simulink model "cpu1"  (R2022b)
settings: Solver=FixedStepDiscrete  StartTime=0.0  StopTime=Inf  RelTol=1e-3  EnableMultiTasking=on
model workspace (MAT data in the model file):
  x = 1
undefined symbols (not defined in the file): C28x, CPU1, CPU2, EALLOW, EDIS
libraries: c2837xDlib x11, dspstat3 x5, c280xlib x4, slpidlib x2, c2802xlib x2, svdutilitieslib x1, dspswit3 x1, idelinklib_common x1
(part 2 of 2)

== matlab function cpu1/Subsystem1/MATLAB Function2 ==
  data: pot_value input; enc input; first_range output; center input; a input; offset input
function first_range = fcn(pot_value,enc,center,a,offset)

    x = center+offset;
    if pot_value < x-(2*a)
        %transition = [-2, -2];
        first_range = -2;
        return
    elseif pot_value < x-a
        transition = [-2, -1];
    elseif pot_value < x
        transition = [-1, 0];
    elseif pot_value < x+a
        transition = [0, 1];
    elseif pot_value < x+(2*a)
        transition = [1, 2];
    else
        %transition = [2, 2];
        first_range = 2;
        return
    end
    distances = abs((x+transition*a)-pot_value);
    if distances(1) <= distances(2)
        index = 1;
    else
        index = 2;
    end
    if distances(index) < 130
        first_range = transition(index);
        return
    end
    %if index == 1
    if enc > 0
        first_range = transition(1);
    else
        first_range = transition(2);
    end
%     else
%         if enc > 0
%             first_range = transition(1);
%         else
%             first_range = transition(2);
%         end

== stateflow chart cpu1/Subsystem/saturation tuned ==
  state state13
    sat = double(delta);
    kp= 0.35;
    if (abs(delta)<=0.5)
    ki=0.18;
    else
    ki=0.12;
    end
    reset = 1;
  state state12
    if delta > 0
    sat = 1;
    else
    sat = -1;
    end
    kp= 0.25;
    reset =0;
  state init
    f20 = 0;
    f15 = 0;
    f10 = 0;
    kp = 0;
    ki = 0;
    kd = 0;
    sat = 0;
  state else
    kp=0;
    sat=0;
    reset =1;
  state state10
    if delta > 0
    sat = 5;
    else
    sat = -5;
    end
    if f20 == 1 && f15==1 && f10==1
    kp = 0.07;
    elseif f20==0 && f15==1 && f10==1
    kp = 0.08;
    elseif f20==0 && f15==0 && f10==1
    kp = 0.08;
    else
    kp= 0.09;
    end
    reset =0;
  state state1
    if delta > 0
    sat = 20;
    else
    sat = -20;
    end
    kp = 0.025;
    f20 = 1;
    reset=0;
  state state9
    if delta > 0
    sat = 15;
    else
    sat = -15;
    end
    if f20 == 1
    kp = 0.03;
    else
    kp = 0.0334;
    end
    f15 = 1;
    reset=0;
  state state8
    if delta > 0
    sat = 10;
    else
    sat = -10;
    end
    if f20 == 1 && f15==1
    kp = 0.04;
    elseif f15==1 && f20==0
    kp = 0.045;
    else
    kp = 0.05;
    end
    f10 = 1;
    reset=0;
  state state11
    if delta > 0
    sat = 2;
    else
    sat = -2;
    end
    if f20 == 1 && f15==1 && f10==1
    kp = 0.15;
    elseif f20==0 && f15==1 && f10==1
    kp = 0.2;
    elseif f20==0 && f15==0 && f10==1
    kp = 0.2;
    else
    kp= 0.22;
    end
    reset =0;
  state13 -> state9 [order 5] : [abs(delta)<20 && abs(delta)>=15]{f20=0,f15=0,f10=0,ki=0}
  state13 -> state10 [order 3] : [abs(delta)>=5 && abs(delta)<10]{f20=0,f15=0,f10=0,ki=0}
  state13 -> state1 [order 6] : [abs(delta)>=20]{f20=0,f15=0,f10=0,ki=0}
  state13 -> state8 [order 4] : [abs(delta)>=10 && abs(delta)<15]{f20=0,f15=0,f10=0,ki=0}
  (junction 7) -> state13 [order 7] : [abs(delta)>=0.04 && abs(delta)<1]
  state8 -> state13 [order 7] : [abs(delta)>=0.04 && abs(delta)<1]
  state13 -> state12 [order 1] : [abs(delta)>=1 && abs(delta)<2]{f20=0,f15=0,f10=0,ki=0}
  state10 -> state13 [order 7] : [abs(delta)>=0.04 && abs(delta)<1]
  state13 -> else [order 7] : [abs(delta)<0.04]{ki=0}
  state9 -> state13 [order 7] : [abs(delta)>=0.04 && abs(delta)<1]
  (junction 7) -> state12 [order 6] : [abs(delta)>=1 && abs(delta)<2]
  state13 -> state11 [order 2] : [abs(delta)>=2 && abs(delta)<5]{f20=0,f15=0,f10=0,ki=0}
  state11 -> state13 [order 7] : [abs(delta)>=0.04 && abs(delta)<1]
  state12 -> state13 [order 7] : [abs(delta)>=0.04 && abs(delta)<1]
  state10 -> state1 [order 3] : [abs(delta)>=20]{f20=0,f15=0,f10=0}
  state12 -> state1 [order 5] : [abs(delta)>=20]
  (default) -> init
  state12 -> state10 [order 2] : [abs(delta)>=5 && abs(delta)<10]
  state1 -> state12 [order 6] : [abs(delta)>=1 && abs(delta)<2]
  state10 -> state12 [order 6] : [abs(delta)>=1 && abs(delta)<2]
  else -> (junction 7) : [~(abs(delta)<0.04)]{f20=0,f15=0,f10=0,reset=0}
  state12 -> else [order 6] : [abs(delta)<0.04]
  state9 -> state12 [order 6] : [abs(delta)>=1 && abs(delta)<2]
  state8 -> state12 [order 6] : [abs(delta)>=1 && abs(delta)<2]
  state1 -> state10 [order 3] : [abs(delta)>=5 && abs(delta)<10]{f20=0}
  state11 -> else [order 1] : [abs(delta)<0.04]
  state12 -> state9 [order 4] : [abs(delta)<20 && abs(delta)>=15]
  state12 -> state8 [order 3] : [abs(delta)>=10 && abs(delta)<15]
  state11 -> state12 [order 6] : [abs(delta)>=1 && abs(delta)<2]
  state12 -> state11 [order 1] : [abs(delta)>=2 && abs(delta)<5]
  state1 -> else [order 4] : [abs(delta)<0.04]
  state9 -> else [order 4] : [abs(delta)<0.04]
  state8 -> else [order 4] : [abs(delta)<0.04]
  state10 -> else [order 4] : [abs(delta)<0.04]
  init -> (junction 7)
  state11 -> state10 [order 2] : [abs(delta)>=5 && abs(delta)<10]{f20=0,f15=0,f10=0}
  state9 -> state10 [order 3] : [abs(delta)>=5 && abs(delta)<10]{f20=0,f15=0,f10=0}
  (junction 7) -> state1 [order 1] : [abs(delta)>=20]
  (junction 7) -> state10 [order 4] : [abs(delta)>=5 && abs(delta)<10]
  (junction 7) -> state11 [order 5] : [abs(delta)>=2 && abs(delta)<5]
  (junction 7) -> state8 [order 2] : [abs(delta)>=10 && abs(delta)<15]
  (junction 7) -> state9 [order 3] : [abs(delta)<20 && abs(delta)>=15]
  state10 -> state11 [order 5] : [abs(delta)>=2 && abs(delta)<5]
  state8 -> state1 [order 1] : [abs(delta)>=20]
  state10 -> state9 [order 2] : [abs(delta)<20 && abs(delta)>=15]{f20=0,f15=0,f10=0}
  state8 -> state10 [order 3] : [abs(delta)>=5 && abs(delta)<10]
  state10 -> state8 [order 1] : [abs(delta)>=10 && abs(delta)<15]{f20=0,f15=0,f10=0}
  state11 -> state1 [order 5] : [abs(delta)>=20]
  state9 -> state1 [order 2] : [abs(delta)>=20]
  state1 -> state9 [order 1] : [abs(delta)<20 && abs(delta)>=15]
  state1 -> state8 [order 2] : [abs(delta)>=10 && abs(delta)<15]{f20=0}
  state1 -> state11 [order 5] : [abs(delta)>=2 && abs(delta)<5]
  state8 -> state9 [order 2] : [abs(delta)<20 && abs(delta)>=15]{f20=0}
  state9 -> state8 [order 1] : [abs(delta)>=10 && abs(delta)<15]
  state11 -> state9 [order 4] : [abs(delta)<20 && abs(delta)>=15]{f20=0,f15=0,f10=0}
  state9 -> state11 [order 5] : [abs(delta)>=2 && abs(delta)<5]
  state8 -> state11 [order 5] : [abs(delta)>=2 && abs(delta)<5]
  state11 -> state8 [order 3] : [abs(delta)>=10 && abs(delta)<15]{f20=0,f15=0,f10=0}
  data: delta input; sat output; kp output; f15 local; f20 local; f10 local; ki output; kd output; v local; reset output

== stateflow chart cpu1/Subsystem/Chart3 ==
  state init
    f15 = 0;
    f10 = 0;
    kp = 0;
    ki = 0;
    kd = 0;
    sat = 0;
  state higherthan15
    if delta > 0
    sat = 15;
    else
    sat = -15;
    end
    kp = 0.0334;
    f15 = 1;
    reset=0;
  state lowerthan15
    reset = 0;
    kp = 0.0334;
    ki = 0.15
    sat = delta;
    reset=1;
    f10 = 1;
  (default) -> init
  init -> (junction 7)
  (junction 7) -> higherthan15 [order 1] : [abs(delta) >15]{f15 =0,f10=0}
  (junction 7) -> lowerthan15 [order 2] : [abs(delta) <15 && abs(delta) >5]{f15 =0,f10=0}
  data: delta input; sat output; kp output; f15 local; f20 local; f10 local; ki output; kd output; v local; reset output

== stateflow chart cpu1/ready ==
  state init
    f15 = 0;
    f10 = 0;
    kp = 0;
    ki = 0;
    kd = 0;
    sat = 0;
  state else
    sat = 0;
    reset = 1;
    kp=0;
    ki=0
  state lowerthan15
    %if f15==0
    %reset=0;
    %end
    sat = delta;
    kp = 0.035;
    kd = 0.0032;
    ki = 0.1;
    reset=1;
    f10 = 1;
  state higherthan15
    ki=0;
    reset=0;
    if delta > 0
    sat = 10;
    else
    sat = -10;
    end
    kp = 0.035;
    kd = 0.0032
    f15 = 1;
  (default) -> init
  (junction 7) -> else [order 3] : [abs(delta) <= 5]
  else -> (junction 7) : [abs(delta) > 5]
  init -> (junction 7)
  higherthan15 -> else [order 2] : [abs(delta) <= 5]{f15=0}
  lowerthan15 -> else [order 2] : [abs(delta) <= 5]
  (junction 7) -> lowerthan15 [order 2] : [abs(delta) <= 10 && abs(delta) > 1]
  (junction 7) -> higherthan15 [order 1] : [abs(delta) >10]
  higherthan15 -> lowerthan15 [order 1] : [abs(delta) <=10  &&   abs(delta) > 1]
  lowerthan15 -> higherthan15 [order 1] : [abs(delta) >10]
  data: delta input single; sat output single; kp output; f15 local; f20 local; f10 local; ki output; kd output; v local; reset output =0

== stateflow chart cpu1/Subsystem/ready1 ==
  state lowerthan1
    sat = delta;
    kp = 0.035;
    kd = 0.0032;
    ki = 0.18;
    reset=1;
  state init
    f15 = 0;
    f10 = 0;
    kp = 0;
    ki = 0;
    kd = 0;
    sat = 0;
  state else
    sat = 0;
    reset = 1;
    kp=0;
    ki=0
  state lowerthan15
    %if f15==0
    %reset=0;
    %end
    sat = delta;
    kp = 0.035;
    kd = 0.0032;
    ki = 0.1;
    reset=1;
    f10 = 1;
  state higherthan15
    ki=0;
    reset=0;
    if delta > 0
    sat = 10;
    else
    sat = -10;
    end
    kp = 0.035;
    kd = 0.0032
    f15 = 1;
  lowerthan1 -> higherthan15 [order 3] : [abs(delta) >10]{ki=0}
  higherthan15 -> lowerthan1 [order 3] : [abs(delta) <= 1 && abs(delta) > 0.04]
  lowerthan1 -> lowerthan15 [order 2] : [abs(delta) <=10  &&   abs(delta) > 1]
  (default) -> init
  (junction 7) -> lowerthan1 [order 3] : [abs(delta) <= 1 && abs(delta) > 0.04]
  lowerthan15 -> lowerthan1 [order 3] : [abs(delta) <= 1 && abs(delta) > 0.04]
  lowerthan1 -> else [order 1] : [abs(delta) <= 0.04]
  (junction 7) -> else [order 4] : [abs(delta) <= 0.04]
  else -> (junction 7) : [abs(delta) > 0.04]
  init -> (junction 7)
  higherthan15 -> else [order 2] : [abs(delta) <= 0.04]{f15=0}
  lowerthan15 -> else [order 2] : [abs(delta) <= 0.04]
  (junction 7) -> lowerthan15 [order 2] : [abs(delta) <= 10 && abs(delta) > 1]
  (junction 7) -> higherthan15 [order 1] : [abs(delta) >10]
  higherthan15 -> lowerthan15 [order 1] : [abs(delta) <=10  &&   abs(delta) > 1]
  lowerthan15 -> higherthan15 [order 1] : [abs(delta) >10]
  data: delta input single; sat output single; kp output; f15 local; f20 local; f10 local; ki output; kd output; v local; reset output =0

== stateflow chart cpu1/Chart4 ==
  state state13
    sat = double(delta);
    kp= 0.3;
    if (abs(delta)<=0.5)
    ki=0.18;
    else
    ki=0.12;
    end
    reset = 1;
  state state12
    if delta > 0
    sat = 1;
    else
    sat = -1;
    end
    kp= 0.25;
    reset =0;
  state else
    kp=0;
    sat=0;
    reset =1;
  state init
    f20 = 0;
    f15 = 0;
    f10 = 0;
    kp = 0;
    ki = 0;
    kd = 0;
    sat = 0;
  state state10
    if delta > 0
    sat = 5;
    else
    sat = -5;
    end
    if f20 == 1 && f15==1 && f10==1
    kp = 0.07;
    elseif f20==0 && f15==1 && f10==1
    kp = 0.08;
    elseif f20==0 && f15==0 && f10==1
    kp = 0.08;
    else
    kp= 0.09;
    end
    reset =0;
  state state1
    if delta > 0
    sat = 20;
    else
    sat = -20;
    end
    kp = 0.025;
    f20 = 1;
    reset=0;
  state state9
    if delta > 0
    sat = 15;
    else
    sat = -15;
    end
    if f20 == 1
    kp = 0.03;
    else
    kp = 0.04;
    end
    f15 = 1;
    reset=0;
  state state8
    if delta > 0
    sat = 10;
    else
    sat = -10;
    end
    if f20 == 1 && f15==1
    kp = 0.04;
    elseif f15==1 && f20==0
    kp = 0.045;
    else
    kp = 0.05;
    end
    f10 = 1;
    reset=0;
  state state11
    if delta > 0
    sat = 2;
    else
    sat = -2;
    end
    if f20 == 1 && f15==1 && f10==1
    kp = 0.15;
    elseif f20==0 && f15==1 && f10==1
    kp = 0.2;
    elseif f20==0 && f15==0 && f10==1
    kp = 0.2;
    else
    kp= 0.22;
    end
    reset =0;
  state13 -> state9 [order 5] : [abs(delta)<20 && abs(delta)>=15]{f20=0,f15=0,f10=0,ki=0}
  state13 -> state10 [order 3] : [abs(delta)>=5 && abs(delta)<10]{f20=0,f15=0,f10=0,ki=0}
  state13 -> state1 [order 6] : [abs(delta)>=20]{f20=0,f15=0,f10=0,ki=0}
  state13 -> state8 [order 4] : [abs(delta)>=10 && abs(delta)<15]{f20=0,f15=0,f10=0,ki=0}
  (junction 7) -> state13 [order 7] : [abs(delta)>=0.04 && abs(delta)<1]
  state8 -> state13 [order 7] : [abs(delta)>=0.04 && abs(delta)<1]
  state13 -> state12 [order 1] : [abs(delta)>=1 && abs(delta)<2]{f20=0,f15=0,f10=0,ki=0}
  state10 -> state13 [order 7] : [abs(delta)>=0.04 && abs(delta)<1]
  state13 -> else [order 7] : [abs(delta)<0.04]{ki=0}
  state9 -> state13 [order 7] : [abs(delta)>=0.04 && abs(delta)<1]
  (junction 7) -> state12 [order 6] : [abs(delta)>=1 && abs(delta)<2]
  state13 -> state11 [order 2] : [abs(delta)>=2 && abs(delta)<5]{f20=0,f15=0,f10=0,ki=0}
  state11 -> state13 [order 7] : [abs(delta)>=0.04 && abs(delta)<1]
  state12 -> state13 [order 7] : [abs(delta)>=0.04 && abs(delta)<1]
  state10 -> state1 [order 3] : [abs(delta)>=20]{f20=0,f15=0,f10=0}
  else -> (junction 7) : [~(abs(delta)<0.04)]{f20=0,f15=0,f10=0,reset=0}
  state12 -> state1 [order 5] : [abs(delta)>=20]
  (default) -> init
  state12 -> state10 [order 2] : [abs(delta)>=5 && abs(delta)<10]
  state12 -> else [order 6] : [abs(delta)<0.04]
  state1 -> state12 [order 6] : [abs(delta)>=1 && abs(delta)<2]
  state10 -> state12 [order 6] : [abs(delta)>=1 && abs(delta)<2]
  state9 -> state12 [order 6] : [abs(delta)>=1 && abs(delta)<2]
  state1 -> else [order 4] : [abs(delta)<0.04]
  state9 -> else [order 4] : [abs(delta)<0.04]
  state8 -> else [order 4] : [abs(delta)<0.04]
  state10 -> else [order 4] : [abs(delta)<0.04]
  state11 -> else [order 1] : [abs(delta)<0.04]
  state8 -> state12 [order 6] : [abs(delta)>=1 && abs(delta)<2]
  state1 -> state10 [order 3] : [abs(delta)>=5 && abs(delta)<10]{f20=0}
  state12 -> state9 [order 4] : [abs(delta)<20 && abs(delta)>=15]
  state12 -> state8 [order 3] : [abs(delta)>=10 && abs(delta)<15]
  state11 -> state12 [order 6] : [abs(delta)>=1 && abs(delta)<2]
  state12 -> state11 [order 1] : [abs(delta)>=2 && abs(delta)<5]
  init -> (junction 7)
  state11 -> state10 [order 2] : [abs(delta)>=5 && abs(delta)<10]{f20=0,f15=0,f10=0}
  state9 -> state10 [order 3] : [abs(delta)>=5 && abs(delta)<10]{f20=0,f15=0,f10=0}
  (junction 7) -> state1 [order 1] : [abs(delta)>=20]
  (junction 7) -> state10 [order 4] : [abs(delta)>=5 && abs(delta)<10]
  (junction 7) -> state11 [order 5] : [abs(delta)>=2 && abs(delta)<5]
  (junction 7) -> state8 [order 2] : [abs(delta)>=10 && abs(delta)<15]
  (junction 7) -> state9 [order 3] : [abs(delta)<20 && abs(delta)>=15]
  state10 -> state11 [order 5] : [abs(delta)>=2 && abs(delta)<5]
  state8 -> state1 [order 1] : [abs(delta)>=20]
  state10 -> state9 [order 2] : [abs(delta)<20 && abs(delta)>=15]{f20=0,f15=0,f10=0}
  state8 -> state10 [order 3] : [abs(delta)>=5 && abs(delta)<10]
  state10 -> state8 [order 1] : [abs(delta)>=10 && abs(delta)<15]{f20=0,f15=0,f10=0}
  state11 -> state1 [order 5] : [abs(delta)>=20]
  state9 -> state1 [order 2] : [abs(delta)>=20]
  state1 -> state9 [order 1] : [abs(delta)<20 && abs(delta)>=15]
  state1 -> state8 [order 2] : [abs(delta)>=10 && abs(delta)<15]{f20=0}
  state1 -> state11 [order 5] : [abs(delta)>=2 && abs(delta)<5]
  state8 -> state9 [order 2] : [abs(delta)<20 && abs(delta)>=15]{f20=0}
  state9 -> state8 [order 1] : [abs(delta)>=10 && abs(delta)<15]
  state11 -> state9 [order 4] : [abs(delta)<20 && abs(delta)>=15]{f20=0,f15=0,f10=0}
  state9 -> state11 [order 5] : [abs(delta)>=2 && abs(delta)<5]
  state8 -> state11 [order 5] : [abs(delta)>=2 && abs(delta)<5]
  state11 -> state8 [order 3] : [abs(delta)>=10 && abs(delta)<15]{f20=0,f15=0,f10=0}
  data: delta input; sat output; kp output; f15 local; f20 local; f10 local; ki output; kd output; v local; reset output

== matlab function cpu1/Subsystem1/MATLAB Function ==
  data: enc input; y output
function y = fcn(enc)
in_min = 0;
in_max = 511;
out_min = -179;
out_max = 180;
y = (enc - in_min) * (out_max - out_min) / (in_max - in_min) + out_min;

end
